simulink model "XecaTurbo_Moist"  (R2023a)
settings: Solver=VariableStepAuto  StartTime=0.0  StopTime=100  RelTol=1e-3  AbsTol=1e-3
PreLoadFcn:
  | omega_TLU = [1000, 1500, 2000, 2500, 3000, 3500];
  | beta_TLU = linspace(0,1,7);
  | 
  | mdot_TLU = [0.1377    0.1304    0.1187    0.1029    0.0854    0.0658    0.0437
  |     0.2310    0.2183    0.1978    0.1688    0.1400    0.1118    0.0750
  |     0.3298    0.3208    0.2987    0.2677    0.2256    0.1774    0.1194
  |     0.4520    0.4260    0.3825    0.3308    0.2745    0.2227    0.1655
  |     0.5542    0.5353    0.4781    0.4230    0.3477    0.2897    0.2211
  |     0.6197    0.5805    0.5198    0.4516    0.3971    0.3555    0.2825];
  | 
  | eta_TLU = [0.7905    0.8025    0.7998    0.7972    0.7932    0.7882    0.7827
  |     0.7993    0.8239    0.8350    0.8379    0.8197    0.8000    0.7809
  |     0.8011    0.8374    0.8632    0.8827    0.8749    0.8394    0.7948
  |     0.8072    0.8520    0.8814    0.9000    0.8676    0.8356    0.7971
  |     0.8076    0.8271    0.8608    0.8766    0.8529    0.8329    0.7992
  |     0.7949    0.8131    0.8296    0.8243    0.8170    0.8085    0.7972];
  | 
  | pr_TLU = [1.0912    1.1795    1.2293    1.2662    1.2928    1.3108    1.3151
  |     1.1484    1.3081    1.3958    1.4707    1.5136    1.5380    1.5456
  |     1.2830    1.4539    1.5943    1.7042    1.7973    1.8582    1.8799
  |     1.5180    1.8034    1.9693    2.0899    2.1662    2.2027    2.2182
  |     1.8359    2.0956    2.3359    2.4668    2.5687    2.6106    2.6224
  |     2.3061    2.6623    2.8585    2.9837    3.0443    3.0714    3.0869];
libraries: nesl_utility x72, fl_lib x52, HVAC_lib x2
(part 1 of 2)
CloseFcn:
  | clear tout simlogCompressorMap
  | clear omega_TLU
  | clear beta_TLU
  | clear mdot_TLU
  | clear pr_TLU
  | clear eta_TLU
Description:
  | Compressor Map
settings Model: Creator=The MathWorks, Inc.  LastModifiedBy=H2FADMIN
settings SolverCC: AutoScaleAbsTol=off  MaxConsecutiveMinStep=25  AlgebraicLoopSolver=TrustRegion  MaxZcPerStep=1
settings DataIOCC: ReturnWorkspaceOutputs=off
settings OptimizationCC: ReuseModelBlockBuffer=off
settings DebuggingCC: UnconnectedInputMsg=warning  UnconnectedOutputMsg=warning  UnconnectedLineMsg=warning  SymbolicDimsDataTypeCodeGenerationDiagnostic=none
settings ModelReferenceCC: EnableRefExpFcnMdlSchedulingChecks=on
settings SFSimCC: CustomCodeUndefinedFunction=UseInterfaceOnly
settings RTWCC: DLArmComputeVersion=19.05
settings SimscapeCC: SimscapeLogType=all  SimscapeLogSimulationStatistics=on  SimscapeLogName=simlogCompressorMap  SimscapeLogDataHistory=10000

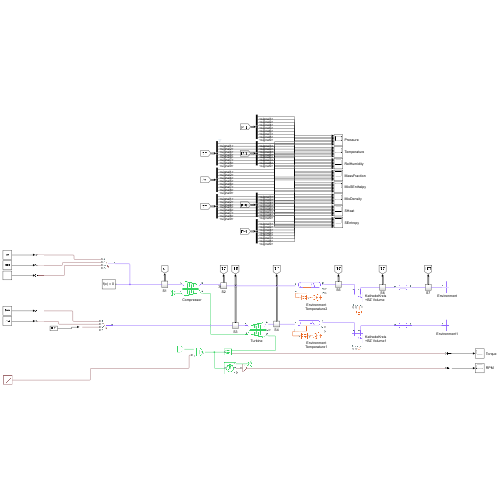
[thumbnail: Simulink's stored preview of the top-level diagram]
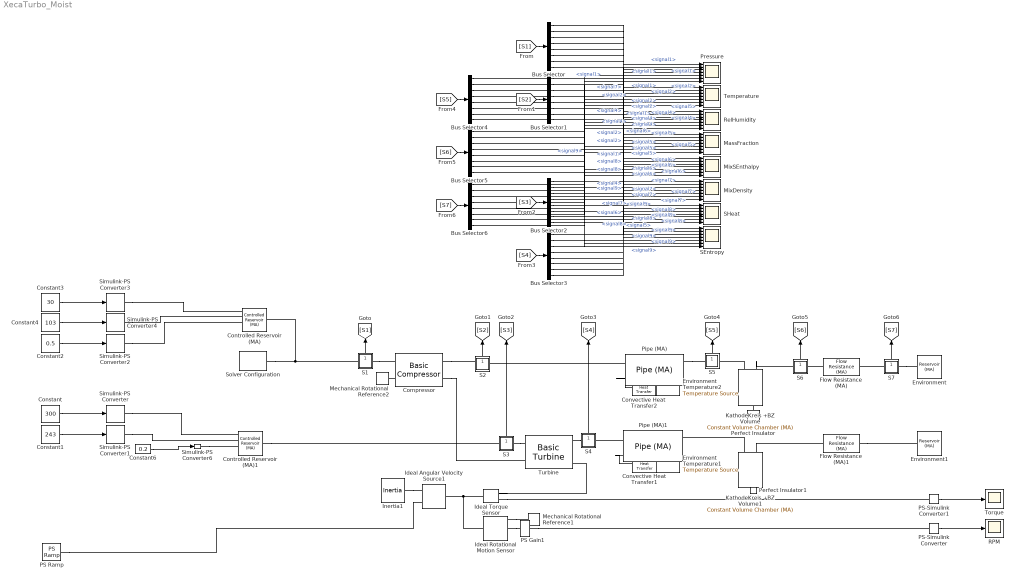
== system XecaTurbo_Moist ==
  Bus Selector{,1..6} (7 alike) : BusSelector  OutputSignals=signal1,signal2,signal4,signal5,signal6,signal7,signal8,signal9
  Compressor : HVAC_lib/Basic Compressor  pr_des=3  mdot_corr_des=.365 kg/s  omega_corr_des=85000 rpm  p_ref=0.101325 MPa  T_ref=288.15 K  RH_ref=0.1  b1=1.5  b2=0.7  b3=0.08  eta_poly=0.95  eta_mech=0.9  area_A=.002 m^2  area_B=.002 m^2
      settings: InternalSimscapePortConfiguration="{\"Bottom\":[],\"Left\":[{\"id\":\"A\",\"label\":\"A\",\"type\":\"foundation.moist_air.moist_air\"},{\"id\":\"C\",\"label\":\"C\",\"type\":\"foundation.mechanical.rotational.rotational\"}],\"Right\":[{\"id\":\"B\",\"label\":\"B\",\"type\":\"foundation.moist_air.moist_air\"},{\"id\":\"R\",\"label\":\"R\",\"type\":\"foundation.mechanical.rotational.rotational\"}],\"Top\":[]}"
  Constant : Constant  Value=300
  Constant1 : Constant  Value=243
  Constant2 : Constant  Value=0.5
  Constant3 : Constant  Value=30
  Constant4 : Constant  Value=103
  Constant6 : Constant  Value=0.2
  Controlled Reservoir (MA) : fl_lib/Moist Air/Elements/Controlled Reservoir (MA)  moisture_spec=foundation.enum.moistureSpec.RelativeHumidity  trace_gas_spec=foundation.enum.trace_gas_spec.mass_fraction  RH_ws=.25  area_A=0.002 m^2  input_error_spec=foundation.enum.input_range_error.limit
      settings: InternalSimscapePortConfiguration="{\"Bottom\":[],\"Left\":[{\"id\":\"A\",\"label\":\"A\",\"type\":\"foundation.moist_air.moist_air\"}],\"Right\":[{\"id\":\"T\",\"label\":\"T\",\"type\":\"input\"},{\"id\":\"P\",\"label\":\"P\",\"type\":\"input\"},{\"id\":\"W\",\"label\":\"W\",\"type\":\"input\"},{\"id\":\"G\",\"label\":\"G\",\"type\":\"input\"}],\"Top\":[]}"
  Controlled Reservoir (MA)1 : fl_lib/Moist Air/Elements/Controlled Reservoir (MA)  moisture_spec=foundation.enum.moistureSpec.RelativeHumidity  trace_gas_spec=foundation.enum.trace_gas_spec.mass_fraction  RH_ws=1  area_A=0.01 m^2  input_error_spec=foundation.enum.input_range_error.limit
      settings: InternalSimscapePortConfiguration="{\"Bottom\":[],\"Left\":[{\"id\":\"A\",\"label\":\"A\",\"type\":\"foundation.moist_air.moist_air\"}],\"Right\":[{\"id\":\"T\",\"label\":\"T\",\"type\":\"input\"},{\"id\":\"P\",\"label\":\"P\",\"type\":\"input\"},{\"id\":\"W\",\"label\":\"W\",\"type\":\"input\"},{\"id\":\"G\",\"label\":\"G\",\"type\":\"input\"}],\"Top\":[]}"
  Convective Heat Transfer1 : fl_lib/Thermal/Thermal Elements/Convective Heat Transfer  thermal_type=foundation.enum.constant_variable.constant  area=.5 m^2  heat_tr_coeff=20 W/(m^2 * K)  min_heat_tr_coeff=1e-3 W/(K*m^2)  T_specify=off  T_priority=None  T=0 K  T_nominal_specify=off  T_nominal_unit=K  T_nominal_value=1  Q_specify=off  Q_priority=None  Q=0 W  Q_nominal_specify=off  Q_nominal_unit=W  Q_nominal_value=1
  Convective Heat Transfer2 : fl_lib/Thermal/Thermal Elements/Convective Heat Transfer  thermal_type=foundation.enum.constant_variable.constant  area=.5 m^2  heat_tr_coeff=20 W/(m^2 * K)  min_heat_tr_coeff=1e-3 W/(K*m^2)  T_specify=off  T_priority=None  T=0 K  T_nominal_specify=off  T_nominal_unit=K  T_nominal_value=1  Q_specify=off  Q_priority=None  Q=0 W  Q_nominal_specify=off  Q_nominal_unit=W  Q_nominal_value=1
  Environment : fl_lib/Moist Air/Elements/Reservoir (MA)  pressure_spec=foundation.enum.pressure_spec.specified  reservoir_pressure=0.103 MPa  temperature_spec=foundation.enum.temperature_spec.specified  reservoir_temperature=20 degC  moisture_spec=foundation.enum.moisture_spec.relative_humidity  reservoir_RH=1  reservoir_x_w=0.01  reservoir_y_w=0.01  reservoir_HR=0.01  reservoir_Tw=287 K  trace_gas_spec=foundation.enum.trace_gas_spec.mole_fraction  reservoir_x_g=0.001  reservoir_y_g=0.1  RH_ws=1  area_A=0.002 m^2
  Environment Temperature1 : fl_lib/Thermal/Thermal Sources/Temperature Source  temperature=20 degC
  Environment Temperature2 : fl_lib/Thermal/Thermal Sources/Temperature Source  temperature=20 degC
  Environment1 : fl_lib/Moist Air/Elements/Reservoir (MA)  pressure_spec=foundation.enum.pressure_spec.specified  reservoir_pressure=0.103 MPa  temperature_spec=foundation.enum.temperature_spec.specified  reservoir_temperature=20 degC  moisture_spec=foundation.enum.moisture_spec.relative_humidity  reservoir_RH=1  reservoir_x_w=0.01  reservoir_y_w=0.01  reservoir_HR=0.01  reservoir_Tw=287 K  trace_gas_spec=foundation.enum.trace_gas_spec.mole_fraction  reservoir_x_g=0.001  reservoir_y_g=0.1  RH_ws=1  area_A=0.002 m^2
  Flow Resistance (MA) : fl_lib/Moist Air/Elements/Flow Resistance (MA)  delta_p_nominal=8 bar  mdot_nominal=.21 kg/s  rho_nominal=3 kg/m^3  area=5.0265482457436691815402294132472e-5 m^2  laminar_fraction=1e-3
  Flow Resistance (MA)1 : fl_lib/Moist Air/Elements/Flow Resistance (MA)  delta_p_nominal=4 bar  mdot_nominal=.21 kg/s  rho_nominal=1.5 kg/m^3  area=5.0265482457436691815402294132472e-5 m^2  laminar_fraction=1e-3
  Ideal Angular Velocity Source1 : fl_lib/Mechanical/Mechanical Sources/Ideal Angular Velocity Source
  Ideal Rotational Motion Sensor : fl_lib/Mechanical/Mechanical Sensors/Ideal Rotational Motion Sensor  reference=foundation.enum.MeasurementReference.difference  acceleration_port=false  velocity_port=true  position_port=true  wrap_angle=false  offset=0 rad
  Ideal Torque Sensor : fl_lib/Mechanical/Mechanical Sensors/Ideal Torque Sensor
  Inertia1 : fl_lib/Mechanical/Rotational Elements/Inertia  inertia=0.03 kg*m^2  num_ports=foundation.enum.numPorts2.one  w_specify=off  w_priority=High  w=0 rad/s  w_nominal_specify=off  w_nominal_unit=rad/s  w_nominal_value=1  t_specify=off  t_priority=None  t=0 N*m  t_nominal_specify=off  t_nominal_unit=N*m  t_nominal_value=1
  KathodeKreis +BZ Volume : fl_lib/Moist Air/Elements/Constant Volume Chamber (MA)  volume=.1 m^3  num_ports=foundation.enum.num_ports.two  area_A=.002 m^2  area_B=.0005 m^2  area_C=0.0005 m^2  area_D=0.01 m^2  RH_ws=1  time_constant=1e-3 s  moisture_trace_gas_source=foundation.enum.moisture_trace_gas_source.controlled  moisture_source_spec=foundation.enum.moisture_source_spec.vapor  moisture_mass_flow=0 kg/s  moisture_temperature_spec=foundation.enum.temperature_spec.atmospheric  moisture_temperature=293.15 K  trace_gas_mass_flow=0 kg/s  trace_gas_temperature_spec=foundation.enum.temperature_spec.atmospheric  trace_gas_temperature=293.15 K  p_I_specify=off  p_I_priority=High  p_I=101.33 kPa  p_I_nominal_specify=off  p_I_nominal_unit=MPa  p_I_nominal_value=1  T_I_specify=off  T_I_priority=High  T_I=45 degC  T_I_nominal_specify=off  T_I_nominal_unit=K  T_I_nominal_value=1  RH_I_specify=off  RH_I_priority=High  RH_I=0.5  RH_I_nominal_specify=off  RH_I_nominal_unit=1  RH_I_nominal_value=1  x_w_I_specify=off  x_w_I_priority=None  x_w_I=0  x_w_I_nominal_specify=off  x_w_I_nominal_unit=1  x_w_I_nominal_value=1  y_w_I_specify=off  y_w_I_priority=None  y_w_I=0  y_w_I_nominal_specify=off  y_w_I_nominal_unit=1  y_w_I_nominal_value=1  HR_I_specify=off  HR_I_priority=None  HR_I=0  HR_I_nominal_specify=off  HR_I_nominal_unit=1  HR_I_nominal_value=1  x_g_I_specify=off  x_g_I_priority=None  x_g_I=0  x_g_I_nominal_specify=off  x_g_I_nominal_unit=1  x_g_I_nominal_value=1  y_g_I_specify=off  y_g_I_priority=High  y_g_I=5e-8  y_g_I_nominal_specify=off  y_g_I_nominal_unit=1  y_g_I_nominal_value=1
      settings: InternalSimscapePortConfiguration="{\"Bottom\":[],\"Left\":[{\"id\":\"A\",\"label\":\"A\",\"type\":\"foundation.moist_air.moist_air\"},{\"id\":\"B\",\"label\":\"B\",\"type\":\"foundation.moist_air.moist_air\"}],\"Right\":[{\"id\":\"W\",\"label\":\"W\",\"type\":\"output\"},{\"id\":\"F\",\"label\":\"F\",\"type\":\"output\"},{\"id\":\"H\",\"label\":\"H\",\"type\":\"foundation.thermal.thermal\"},{\"id\":\"S\",\"label\":\"S\",\"type\":\"foundation.moist_air.moist_air_source\"}],\"Top\":[]}"
  KathodeKreis +BZ Volume1 : fl_lib/Moist Air/Elements/Constant Volume Chamber (MA)  volume=.1 m^3  num_ports=foundation.enum.num_ports.two  area_A=.002 m^2  area_B=.002 m^2  area_C=0.0005 m^2  area_D=0.01 m^2  RH_ws=1  time_constant=1e-3 s  moisture_trace_gas_source=foundation.enum.moisture_trace_gas_source.controlled  moisture_source_spec=foundation.enum.moisture_source_spec.vapor  moisture_mass_flow=0 kg/s  moisture_temperature_spec=foundation.enum.temperature_spec.atmospheric  moisture_temperature=293.15 K  trace_gas_mass_flow=0 kg/s  trace_gas_temperature_spec=foundation.enum.temperature_spec.atmospheric  trace_gas_temperature=293.15 K  p_I_specify=off  p_I_priority=High  p_I=101.33 kPa  p_I_nominal_specify=off  p_I_nominal_unit=MPa  p_I_nominal_value=1  T_I_specify=on  T_I_priority=High  T_I=45 degC  T_I_nominal_specify=off  T_I_nominal_unit=K  T_I_nominal_value=1  RH_I_specify=off  RH_I_priority=High  RH_I=0.5  RH_I_nominal_specify=off  RH_I_nominal_unit=1  RH_I_nominal_value=1  x_w_I_specify=off  x_w_I_priority=None  x_w_I=0  x_w_I_nominal_specify=off  x_w_I_nominal_unit=1  x_w_I_nominal_value=1  y_w_I_specify=off  y_w_I_priority=None  y_w_I=0  y_w_I_nominal_specify=off  y_w_I_nominal_unit=1  y_w_I_nominal_value=1  HR_I_specify=off  HR_I_priority=None  HR_I=0  HR_I_nominal_specify=off  HR_I_nominal_unit=1  HR_I_nominal_value=1  x_g_I_specify=off  x_g_I_priority=None  x_g_I=0  x_g_I_nominal_specify=off  x_g_I_nominal_unit=1  x_g_I_nominal_value=1  y_g_I_specify=off  y_g_I_priority=High  y_g_I=5e-8  y_g_I_nominal_specify=off  y_g_I_nominal_unit=1  y_g_I_nominal_value=1
      settings: InternalSimscapePortConfiguration="{\"Bottom\":[],\"Left\":[{\"id\":\"A\",\"label\":\"A\",\"type\":\"foundation.moist_air.moist_air\"},{\"id\":\"B\",\"label\":\"B\",\"type\":\"foundation.moist_air.moist_air\"}],\"Right\":[{\"id\":\"W\",\"label\":\"W\",\"type\":\"output\"},{\"id\":\"F\",\"label\":\"F\",\"type\":\"output\"},{\"id\":\"H\",\"label\":\"H\",\"type\":\"foundation.thermal.thermal\"},{\"id\":\"S\",\"label\":\"S\",\"type\":\"foundation.moist_air.moist_air_source\"}],\"Top\":[]}"
  MassFraction : Scope  NumInputPorts=7
  Mechanical Rotational Reference1 : fl_lib/Mechanical/Rotational Elements/Mechanical Rotational Reference
  Mechanical Rotational Reference2 : fl_lib/Mechanical/Rotational Elements/Mechanical Rotational Reference
  MixDensity : Scope  NumInputPorts=7
  MixSEnthalpy : Scope  NumInputPorts=7
  PS Gain1 : fl_lib/Physical Signals/Functions/PS Gain  gain=1/(0.1047198*1000)
  PS Ramp : fl_lib/Physical Signals/Sources/PS Ramp  slope=(85000-31000)/90 rpm/s  start_time=10 s  initial_output=31000 rpm
  PS-Simulink Converter : nesl_utility/PS-Simulink Converter  PhysicalDomain=network_engine_domain  SubClassName=ps_output  LeftPortType=input  RightPortType=output  PseudoPeriodic=off  Frequencies=[]  VectorFormat=inherit  Unit=inherit  AffineConversion=off
  PS-Simulink Converter1 : nesl_utility/PS-Simulink Converter  PhysicalDomain=network_engine_domain  SubClassName=ps_output  LeftPortType=input  RightPortType=output  PseudoPeriodic=off  Frequencies=[]  VectorFormat=inherit  Unit=inherit  AffineConversion=off
  Perfect Insulator : fl_lib/Thermal/Thermal Elements/Perfect Insulator  T_specify=off  T_priority=None  T=293.15 K  T_nominal_specify=off  T_nominal_unit=K  T_nominal_value=1
  Perfect Insulator1 : fl_lib/Thermal/Thermal Elements/Perfect Insulator  T_specify=off  T_priority=None  T=293.15 K  T_nominal_specify=off  T_nominal_unit=K  T_nominal_value=1
  Pipe (MA) : fl_lib/Moist Air/Elements/Pipe (MA)  length=1 m  area=.002 m^2  Dh=.1 m  length_add=1 m  roughness=15e-5 m  Re_lam=2000  Re_tur=4000  shape_factor=64  Nu_lam=3.66  wall_condensation=simscape.enum.onoff.off  RH_ws=1  time_constant=1e-3 s  moisture_trace_gas_source=foundation.enum.moisture_trace_gas_source.none  moisture_source_spec=foundation.enum.moisture_source_spec.vapor  moisture_mass_flow=0 kg/s  moisture_temperature_spec=foundation.enum.temperature_spec.atmospheric  moisture_temperature=293.15 K  trace_gas_mass_flow=0 kg/s  trace_gas_temperature_spec=foundation.enum.temperature_spec.atmospheric  trace_gas_temperature=293.15 K  p_I_specify=off  p_I_priority=High  p_I=0.103 MPa  p_I_nominal_specify=off  p_I_nominal_unit=MPa  p_I_nominal_value=1  T_I_specify=off  T_I_priority=High  T_I=20 degC  T_I_nominal_specify=off  T_I_nominal_unit=K  T_I_nominal_value=1  RH_I_specify=off  RH_I_priority=High  RH_I=1  RH_I_nominal_specify=off  RH_I_nominal_unit=1  RH_I_nominal_value=1  x_w_I_specify=off  x_w_I_priority=None  x_w_I=0  x_w_I_nominal_specify=off  x_w_I_nominal_unit=1  x_w_I_nominal_value=1  y_w_I_specify=off  y_w_I_priority=None  y_w_I=0  y_w_I_nominal_specify=off  y_w_I_nominal_unit=1  y_w_I_nominal_value=1  HR_I_specify=off  HR_I_priority=None  HR_I=0  HR_I_nominal_specify=off  HR_I_nominal_unit=1  HR_I_nominal_value=1  x_g_I_specify=off  x_g_I_priority=None  x_g_I=0  x_g_I_nominal_specify=off  x_g_I_nominal_unit=1  x_g_I_nominal_value=1  y_g_I_specify=off  y_g_I_priority=High  y_g_I=0.1  y_g_I_nominal_specify=off  y_g_I_nominal_unit=1  y_g_I_nominal_value=1
  Pipe (MA)1 : fl_lib/Moist Air/Elements/Pipe (MA)  length=1 m  area=.002 m^2  Dh=.1 m  length_add=1 m  roughness=15e-5 m  Re_lam=2000  Re_tur=4000  shape_factor=64  Nu_lam=3.66  wall_condensation=simscape.enum.onoff.off  RH_ws=1  time_constant=1e-3 s  moisture_trace_gas_source=foundation.enum.moisture_trace_gas_source.none  moisture_source_spec=foundation.enum.moisture_source_spec.vapor  moisture_mass_flow=0 kg/s  moisture_temperature_spec=foundation.enum.temperature_spec.atmospheric  moisture_temperature=293.15 K  trace_gas_mass_flow=0 kg/s  trace_gas_temperature_spec=foundation.enum.temperature_spec.atmospheric  trace_gas_temperature=293.15 K  p_I_specify=off  p_I_priority=High  p_I=0.103 MPa  p_I_nominal_specify=off  p_I_nominal_unit=MPa  p_I_nominal_value=1  T_I_specify=off  T_I_priority=High  T_I=20 degC  T_I_nominal_specify=off  T_I_nominal_unit=K  T_I_nominal_value=1  RH_I_specify=off  RH_I_priority=High  RH_I=1  RH_I_nominal_specify=off  RH_I_nominal_unit=1  RH_I_nominal_value=1  x_w_I_specify=off  x_w_I_priority=None  x_w_I=0  x_w_I_nominal_specify=off  x_w_I_nominal_unit=1  x_w_I_nominal_value=1  y_w_I_specify=off  y_w_I_priority=None  y_w_I=0  y_w_I_nominal_specify=off  y_w_I_nominal_unit=1  y_w_I_nominal_value=1  HR_I_specify=off  HR_I_priority=None  HR_I=0  HR_I_nominal_specify=off  HR_I_nominal_unit=1  HR_I_nominal_value=1  x_g_I_specify=off  x_g_I_priority=None  x_g_I=0  x_g_I_nominal_specify=off  x_g_I_nominal_unit=1  x_g_I_nominal_value=1  y_g_I_specify=off  y_g_I_priority=High  y_g_I=0.1  y_g_I_nominal_specify=off  y_g_I_nominal_unit=1  y_g_I_nominal_value=1
  Pressure : Scope  NumInputPorts=7
  RPM : Scope
  RelHumidity : Scope  NumInputPorts=7
  S1 : Subsystem
      settings: PortSchema="{\"entries\":[{\"content\":{\"sides\":[{\"content\":{\"connectorIds\":[\"LConn1\"]},\"type\":\"ConnectorPlacement.EquallySpacedRectSide\",\"uuid\":\"254e2835-1051-41ce-ae2c-1054ced4b7e5\"},{\"content\":{\"connectorIds\":[\"RConn1\"],\"side\":\"RIGHT\"},\"type\":\"ConnectorPlacement.EquallySpacedRectSide\",\"uuid\":\"319e61c8-525d-4586-8cb8-060a189dde36\"},{\"content\":{\"connectorIds\":[\"Out1\"],\"side\":\"TOP\"},\"type\":\"ConnectorPlacement.EquallySpacedRectSide\",\"uuid\":\"621e15c0-a15c-4528-a2f1-5cf6f15ed99c\"}]},\"type\":\"ConnectorPlacement.EquallySpacedConnector\",\"uuid\":\"0cef8054-f5e2-4319-9020-84a4d4054be4\"}],\"packageUris\":[\"http://schema.mathworks.com/mf0/Connector/R2020b\"],\"version\":\"1.0\"}"
  S2 : Subsystem
      settings: PortSchema="{\"entries\":[{\"content\":{\"sides\":[{\"content\":{\"connectorIds\":[\"LConn1\",\"LConn2\",\"LConn3\"]},\"type\":\"ConnectorPlacement.EquallySpacedRectSide\",\"uuid\":\"2c3dff3d-006a-434f-af42-26af1dfa59bd\"},{\"content\":{\"connectorIds\":[\"RConn1\"],\"side\":\"RIGHT\"},\"type\":\"ConnectorPlacement.EquallySpacedRectSide\",\"uuid\":\"5c8d4e8e-dace-4a30-a25f-c68d34fe03f2\"},{\"content\":{\"connectorIds\":[\"Out1\"],\"side\":\"TOP\"},\"type\":\"ConnectorPlacement.EquallySpacedRectSide\",\"uuid\":\"01211e8f-380a-4edd-8d10-28a378ec8de7\"}]},\"type\":\"ConnectorPlacement.EquallySpacedConnector\",\"uuid\":\"cc392eb8-3a05-4333-a2d0-35104579f5e5\"}],\"packageUris\":[\"http://schema.mathworks.com/mf0/Connector/R2020b\"],\"version\":\"1.0\"}"
  S3 : Subsystem
      settings: PortSchema="{\"entries\":[{\"content\":{\"sides\":[{\"content\":{\"connectorIds\":[\"LConn1\"]},\"type\":\"ConnectorPlacement.EquallySpacedRectSide\",\"uuid\":\"254e2835-1051-41ce-ae2c-1054ced4b7e5\"},{\"content\":{\"connectorIds\":[\"RConn1\"],\"side\":\"RIGHT\"},\"type\":\"ConnectorPlacement.EquallySpacedRectSide\",\"uuid\":\"319e61c8-525d-4586-8cb8-060a189dde36\"},{\"content\":{\"connectorIds\":[\"Out1\"],\"side\":\"TOP\"},\"type\":\"ConnectorPlacement.EquallySpacedRectSide\",\"uuid\":\"621e15c0-a15c-4528-a2f1-5cf6f15ed99c\"}]},\"type\":\"ConnectorPlacement.EquallySpacedConnector\",\"uuid\":\"0cef8054-f5e2-4319-9020-84a4d4054be4\"}],\"packageUris\":[\"http://schema.mathworks.com/mf0/Connector/R2020b\"],\"version\":\"1.0\"}"
  S4 : Subsystem
      settings: PortSchema="{\"entries\":[{\"content\":{\"sides\":[{\"content\":{\"connectorIds\":[\"LConn1\"]},\"type\":\"ConnectorPlacement.EquallySpacedRectSide\",\"uuid\":\"254e2835-1051-41ce-ae2c-1054ced4b7e5\"},{\"content\":{\"connectorIds\":[\"RConn1\"],\"side\":\"RIGHT\"},\"type\":\"ConnectorPlacement.EquallySpacedRectSide\",\"uuid\":\"319e61c8-525d-4586-8cb8-060a189dde36\"},{\"content\":{\"connectorIds\":[\"Out1\"],\"side\":\"TOP\"},\"type\":\"ConnectorPlacement.EquallySpacedRectSide\",\"uuid\":\"621e15c0-a15c-4528-a2f1-5cf6f15ed99c\"}]},\"type\":\"ConnectorPlacement.EquallySpacedConnector\",\"uuid\":\"0cef8054-f5e2-4319-9020-84a4d4054be4\"}],\"packageUris\":[\"http://schema.mathworks.com/mf0/Connector/R2020b\"],\"version\":\"1.0\"}"
  S5 : Subsystem
      settings: PortSchema="{\"entries\":[{\"content\":{\"sides\":[{\"content\":{\"connectorIds\":[\"LConn1\"]},\"type\":\"ConnectorPlacement.EquallySpacedRectSide\",\"uuid\":\"254e2835-1051-41ce-ae2c-1054ced4b7e5\"},{\"content\":{\"connectorIds\":[\"RConn1\"],\"side\":\"RIGHT\"},\"type\":\"ConnectorPlacement.EquallySpacedRectSide\",\"uuid\":\"319e61c8-525d-4586-8cb8-060a189dde36\"},{\"content\":{\"connectorIds\":[\"Out1\"],\"side\":\"TOP\"},\"type\":\"ConnectorPlacement.EquallySpacedRectSide\",\"uuid\":\"621e15c0-a15c-4528-a2f1-5cf6f15ed99c\"}]},\"type\":\"ConnectorPlacement.EquallySpacedConnector\",\"uuid\":\"0cef8054-f5e2-4319-9020-84a4d4054be4\"}],\"packageUris\":[\"http://schema.mathworks.com/mf0/Connector/R2020b\"],\"version\":\"1.0\"}"
  S6 : Subsystem
      settings: PortSchema="{\"entries\":[{\"content\":{\"sides\":[{\"content\":{\"connectorIds\":[\"LConn1\"]},\"type\":\"ConnectorPlacement.EquallySpacedRectSide\",\"uuid\":\"254e2835-1051-41ce-ae2c-1054ced4b7e5\"},{\"content\":{\"connectorIds\":[\"RConn1\"],\"side\":\"RIGHT\"},\"type\":\"ConnectorPlacement.EquallySpacedRectSide\",\"uuid\":\"319e61c8-525d-4586-8cb8-060a189dde36\"},{\"content\":{\"connectorIds\":[\"Out1\"],\"side\":\"TOP\"},\"type\":\"ConnectorPlacement.EquallySpacedRectSide\",\"uuid\":\"621e15c0-a15c-4528-a2f1-5cf6f15ed99c\"}]},\"type\":\"ConnectorPlacement.EquallySpacedConnector\",\"uuid\":\"0cef8054-f5e2-4319-9020-84a4d4054be4\"}],\"packageUris\":[\"http://schema.mathworks.com/mf0/Connector/R2020b\"],\"version\":\"1.0\"}"
  S7 : Subsystem
      settings: PortSchema="{\"entries\":[{\"content\":{\"sides\":[{\"content\":{\"connectorIds\":[\"LConn1\"]},\"type\":\"ConnectorPlacement.EquallySpacedRectSide\",\"uuid\":\"254e2835-1051-41ce-ae2c-1054ced4b7e5\"},{\"content\":{\"connectorIds\":[\"RConn1\"],\"side\":\"RIGHT\"},\"type\":\"ConnectorPlacement.EquallySpacedRectSide\",\"uuid\":\"319e61c8-525d-4586-8cb8-060a189dde36\"},{\"content\":{\"connectorIds\":[\"Out1\"],\"side\":\"TOP\"},\"type\":\"ConnectorPlacement.EquallySpacedRectSide\",\"uuid\":\"621e15c0-a15c-4528-a2f1-5cf6f15ed99c\"}]},\"type\":\"ConnectorPlacement.EquallySpacedConnector\",\"uuid\":\"0cef8054-f5e2-4319-9020-84a4d4054be4\"}],\"packageUris\":[\"http://schema.mathworks.com/mf0/Connector/R2020b\"],\"version\":\"1.0\"}"
  SEntropy : Scope  NumInputPorts=7
  SHeat : Scope  NumInputPorts=7
  Simulink-PS Converter : nesl_utility/Simulink-PS Converter  PhysicalDomain=network_engine_domain  SubClassName=ps_input  LeftPortType=input  RightPortType=output  PseudoPeriodic=off  Frequencies=[]  NoiseDistribution=none  NoiseParameters=[]  Unit=degC  AffineConversion=off  FilteringAndDerivatives=provide  SimscapeFilterOrder=1  InputFilterTimeConstant=0.001  UdotUserProvided=0
  Simulink-PS Converter1 : nesl_utility/Simulink-PS Converter  PhysicalDomain=network_engine_domain  SubClassName=ps_input  LeftPortType=input  RightPortType=output  PseudoPeriodic=off  Frequencies=[]  NoiseDistribution=none  NoiseParameters=[]  Unit=kPa  AffineConversion=off  FilteringAndDerivatives=provide  SimscapeFilterOrder=1  InputFilterTimeConstant=0.001  UdotUserProvided=0
  Simulink-PS Converter2 : nesl_utility/Simulink-PS Converter  PhysicalDomain=network_engine_domain  SubClassName=ps_input  LeftPortType=input  RightPortType=output  PseudoPeriodic=off  Frequencies=[]  NoiseDistribution=none  NoiseParameters=[]  Unit=1  AffineConversion=off  FilteringAndDerivatives=provide  SimscapeFilterOrder=1  InputFilterTimeConstant=0.001  UdotUserProvided=0
  Simulink-PS Converter3 : nesl_utility/Simulink-PS Converter  PhysicalDomain=network_engine_domain  SubClassName=ps_input  LeftPortType=input  RightPortType=output  PseudoPeriodic=off  Frequencies=[]  NoiseDistribution=none  NoiseParameters=[]  Unit=degC  AffineConversion=off  FilteringAndDerivatives=provide  SimscapeFilterOrder=1  InputFilterTimeConstant=0.001  UdotUserProvided=0
  Simulink-PS Converter4 : nesl_utility/Simulink-PS Converter  PhysicalDomain=network_engine_domain  SubClassName=ps_input  LeftPortType=input  RightPortType=output  PseudoPeriodic=off  Frequencies=[]  NoiseDistribution=none  NoiseParameters=[]  Unit=kPa  AffineConversion=off  FilteringAndDerivatives=provide  SimscapeFilterOrder=1  InputFilterTimeConstant=0.001  UdotUserProvided=0
  Simulink-PS Converter6 : nesl_utility/Simulink-PS Converter  PhysicalDomain=network_engine_domain  SubClassName=ps_input  LeftPortType=input  RightPortType=output  PseudoPeriodic=off  Frequencies=[]  NoiseDistribution=none  NoiseParameters=[]  Unit=1  AffineConversion=off  FilteringAndDerivatives=provide  SimscapeFilterOrder=1  InputFilterTimeConstant=0.001  UdotUserProvided=0
  Solver Configuration : nesl_utility/Solver Configuration  PhysicalDomain=network_engine_domain  SubClassName=solver  LeftPortType=input  RightPortType=generic  Tones=[]  Harmonics=[]  SimulateNoise=off  Profile=off  UseLocalSampling=off  EnableSwitchedLinearOptims=on  FrequencyDomain=off  UseCCode=off  RelTol=0.001  AbsTol=0.001  MinStep=1e-09  ToWorkspace=off  RevertToSquareIcSolve=off  NumHomotopyIterations=100  PhasorMode=off  PhasorModeNumHarmonics=1  ConsistencySolver=NEWTON_XTOL_AFTER_FTOL  IndexReductionMethod=DerivativeReplacement  DoDC=off  ResidualTolerance=1e-09  ConsistencyTolSource=GLOBAL  ConsistencyAbsTol=0.001  ConsistencyRelTol=0.001  ConsistencyTolFactor=0.001  UseLocalSolver=on  LocalSolverChoice=NE_BACKWARD_EULER_ADVANCER  ResolveIndetEquations=on  FunctionEvalNumThread=1  LocalSolverSampleTime=0.001  DoFixedCost=on  MaxNonlinIter=3  MaxModeIter=2  ComputeImpulses=off  ImpulseIterations=2  LinearAlgebra=auto  LinearAlgebraNumThread=0  EquationFormulation=NE_TIME_EF  DelaysMemoryBudget=1024  AutomaticFiltering=on  FilteringTimeConstant=0.001  PartitionStorageMethod=AS_NEEDED  PartitionMemoryBudget=1024  PartitionMethod=ROBUST
  Temperature : Scope  NumInputPorts=7
  Torque : Scope
  Turbine : HVAC_lib/Basic Turbine  pr_des=0.2  mdot_corr_des=0.22 kg/s  p_ref=0.101325 MPa  T_ref=288.15 K  RH_ref=0  eta_poly=0.92  eta_mech=0.98  area_A=.002 m^2  area_B=.002 m^2  RH_ws=1
      settings: InternalSimscapePortConfiguration="{\"Bottom\":[],\"Left\":[{\"id\":\"A\",\"label\":\"A\",\"type\":\"foundation.moist_air.moist_air\"},{\"id\":\"R\",\"label\":\"R\",\"type\":\"foundation.mechanical.rotational.rotational\"}],\"Right\":[{\"id\":\"B\",\"label\":\"B\",\"type\":\"foundation.moist_air.moist_air\"},{\"id\":\"W\",\"label\":\"W\",\"type\":\"output\"},{\"id\":\"C\",\"label\":\"C\",\"type\":\"foundation.mechanical.rotational.rotational\"}],\"Top\":[]}"
  wires:
  Bus Selector3/2 -> Temperature/4  "<signal2>"
  Bus Selector2/8 -> SEntropy/3  "<signal9>"
  [S1] -> Bus Selector/1
  Bus Selector3/4 -> MassFraction/4  "<signal5>"
  Bus Selector1/7 -> SHeat/2  "<signal8>"
  Bus Selector1/6 -> MixDensity/2  "<signal7>"
  [S2] -> Bus Selector1/1
  Bus Selector4/2 -> Temperature/6  "<signal2>"
  Bus Selector5/3 -> RelHumidity/5  "<signal4>"
  PS-Simulink Converter/1 -> RPM/1
  [S3] -> Bus Selector2/1
  Bus Selector5/4 -> MassFraction/5  "<signal5>"
  [S6] -> Bus Selector5/1
  [S4] -> Bus Selector3/1
  [S5] -> Bus Selector4/1
  [S7] -> Bus Selector6/1
  Bus Selector6/1 -> Pressure/7  "<signal1>"
  Bus Selector1/2 -> Temperature/2  "<signal2>"
  Bus Selector2/5 -> MixSEnthalpy/3  "<signal6>"
  S1/1(Outport) -> [S1]
  Bus Selector/2 -> Temperature/1  "<signal2>"
  Bus Selector/1 -> Pressure/1  "<signal1>"
  Bus Selector/4 -> RelHumidity/1  "<signal5>"
  Bus Selector5/1 -> Pressure/5  "<signal1>"
  Bus Selector/3 -> MassFraction/1  "<signal4>"
  Bus Selector1/5 -> MixSEnthalpy/2  "<signal6>"
  Bus Selector/5 -> MixSEnthalpy/1  "<signal6>"
  Bus Selector/8 -> SEntropy/1  "<signal9>"
  Bus Selector/6 -> MixDensity/1  "<signal7>"
  Bus Selector/7 -> SHeat/1  "<signal8>"
  Bus Selector1/1 -> Pressure/2  "<signal1>"
  Bus Selector4/4 -> MassFraction/6  "<signal5>"
  Bus Selector5/6 -> MixDensity/5  "<signal7>"
  Bus Selector3/7 -> SHeat/4  "<signal8>"
  Bus Selector1/3 -> RelHumidity/2  "<signal4>"
  Bus Selector1/4 -> MassFraction/2  "<signal5>"
  Bus Selector2/2 -> Temperature/3  "<signal2>"
  Bus Selector1/8 -> SEntropy/2  "<signal9>"
  Bus Selector2/1 -> Pressure/3  "<signal1>"
  Bus Selector2/3 -> RelHumidity/3  "<signal4>"
  Bus Selector2/4 -> MassFraction/3  "<signal5>"
  Bus Selector2/6 -> MixDensity/3  "<signal7>"
  Bus Selector2/7 -> SHeat/3  "<signal8>"
  Bus Selector3/1 -> Pressure/4  "<signal1>"
  Bus Selector4/3 -> RelHumidity/6  "<signal4>"
  Bus Selector3/3 -> RelHumidity/4  "<signal4>"
  Bus Selector3/5 -> MixSEnthalpy/4  "<signal6>"
  Bus Selector3/6 -> MixDensity/4  "<signal7>"
  Bus Selector3/8 -> SEntropy/4  "<signal9>"
  Bus Selector4/1 -> Pressure/6  "<signal1>"
  Bus Selector5/2 -> Temperature/5  "<signal2>"
  Bus Selector5/5 -> MixSEnthalpy/5  "<signal6>"
  Bus Selector4/5 -> MixSEnthalpy/6  "<signal6>"
  Bus Selector5/7 -> SHeat/5  "<signal8>"
  Bus Selector4/6 -> MixDensity/6  "<signal7>"
  Bus Selector5/8 -> SEntropy/5  "<signal9>"
  Bus Selector4/7 -> SHeat/6  "<signal8>"
  Bus Selector4/8 -> SEntropy/6  "<signal9>"
  Bus Selector6/2 -> Temperature/7  "<signal2>"
  Bus Selector6/3 -> RelHumidity/7  "<signal4>"
  Bus Selector6/4 -> MassFraction/7  "<signal5>"
  Bus Selector6/5 -> MixSEnthalpy/7  "<signal6>"
  Bus Selector6/6 -> MixDensity/7  "<signal7>"
  Bus Selector6/7 -> SHeat/7  "<signal8>"
  Bus Selector6/8 -> SEntropy/7  "<signal9>"
  PS-Simulink Converter1/1 -> Torque/1
  S2/1(Outport) -> [S2]
  S3/1(Outport) -> [S3]
  S4/1(Outport) -> [S4]
  S5/1(Outport) -> [S5]
  S6/1(Outport) -> [S6]
  S7/1(Outport) -> [S7]
  Constant2/1 -> Simulink-PS Converter2/1
  Constant/1 -> Simulink-PS Converter/1
  Constant1/1 -> Simulink-PS Converter1/1
  Constant6/1 -> Simulink-PS Converter6/1
  Constant4/1 -> Simulink-PS Converter4/1
  Constant3/1 -> Simulink-PS Converter3/1
  connections:
  Ideal Rotational Motion Sensor/RConn2 -- PS Gain1/LConn1
  Ideal Rotational Motion Sensor/RConn1 -- Mechanical Rotational Reference1/LConn1
  Ideal Torque Sensor/RConn2 -- PS-Simulink Converter1/LConn1
  Inertia1/LConn1 -- Ideal Angular Velocity Source1/RConn2
  Ideal Rotational Motion Sensor/LConn1 -- Ideal Torque Sensor/LConn1 -- Ideal Angular Velocity Source1/LConn1
  PS Ramp/RConn1 -- Ideal Angular Velocity Source1/RConn1
  Solver Configuration/RConn1 -- S1/LConn1 -- Controlled Reservoir (MA)/LConn1
  PS Gain1/RConn1 -- PS-Simulink Converter/LConn1
  S1/RConn1 -- Compressor/LConn1
  KathodeKreis +BZ Volume/LConn2 -- S6/LConn1
  Compressor/RConn2 -- Turbine/LConn2
  Compressor/RConn1 -- S2/LConn1
  Controlled Reservoir (MA)1/LConn1 -- S3/LConn1
  S3/RConn1 -- Turbine/LConn1
  Turbine/RConn1 -- S4/LConn1
  Ideal Torque Sensor/RConn1 -- Turbine/RConn3
  KathodeKreis +BZ Volume/LConn1 -- S5/RConn1
  Pipe (MA)/LConn2 -- Convective Heat Transfer2/LConn1
  Flow Resistance (MA)/LConn1 -- S6/RConn1
  Convective Heat Transfer2/RConn1 -- Environment Temperature2/LConn1
  Pipe (MA)/RConn1 -- S5/LConn1
  Simulink-PS Converter3/RConn1 -- Controlled Reservoir (MA)/RConn1
  Simulink-PS Converter4/RConn1 -- Controlled Reservoir (MA)/RConn2
  Simulink-PS Converter2/RConn1 -- Controlled Reservoir (MA)/RConn3
  Simulink-PS Converter6/RConn1 -- Controlled Reservoir (MA)1/RConn3
  S7/LConn1 -- Flow Resistance (MA)/RConn1
  S7/RConn1 -- Environment/LConn1
  Perfect Insulator/LConn1 -- KathodeKreis +BZ Volume/RConn3
  Pipe (MA)/LConn1 -- S2/RConn1
  Perfect Insulator1/LConn1 -- KathodeKreis +BZ Volume1/RConn3
  Convective Heat Transfer1/RConn1 -- Environment Temperature1/LConn1
  Flow Resistance (MA)1/RConn1 -- Environment1/LConn1
  KathodeKreis +BZ Volume1/LConn2 -- Flow Resistance (MA)1/LConn1
  Pipe (MA)1/LConn1 -- S4/RConn1
  Pipe (MA)1/LConn2 -- Convective Heat Transfer1/LConn1
  KathodeKreis +BZ Volume1/LConn1 -- Pipe (MA)1/RConn1
  Simulink-PS Converter/RConn1 -- Controlled Reservoir (MA)1/RConn1
  Simulink-PS Converter1/RConn1 -- Controlled Reservoir (MA)1/RConn2
  Mechanical Rotational Reference2/LConn1 -- Compressor/LConn2

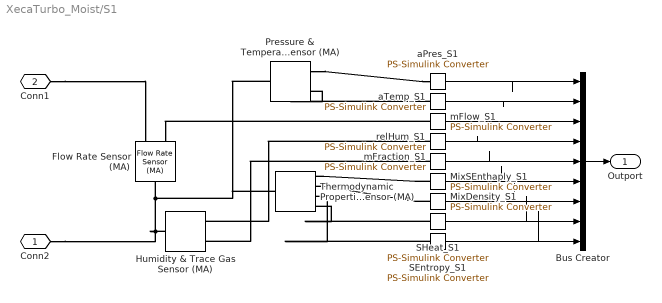
== system XecaTurbo_Moist/S1 ==
  Bus Creator : BusCreator  Inputs=9
  Flow Rate Sensor (MA) : fl_lib/Moist Air/Sensors/Flow Rate Sensor (MA)  mass_flow_measure=true  volumetric_flow_measure=false  volumetric_flow_conditions=foundation.enum.volumetric_flow_conditions.actual  p_std=0.101325 MPa  T_std=20 degC  RH_std=0.65  energy_flow_measure=false  vapor_flow_measure=false  gas_flow_measure=false
      settings: InternalSimscapePortConfiguration="{\"Bottom\":[],\"Left\":[{\"id\":\"A\",\"label\":\"A\",\"type\":\"foundation.moist_air.moist_air\"}],\"Right\":[{\"id\":\"B\",\"label\":\"B\",\"type\":\"foundation.moist_air.moist_air\"},{\"id\":\"M\",\"label\":\"M\",\"type\":\"output\"}],\"Top\":[]}"
  Humidity & Trace Gas Sensor (MA) : fl_lib/Moist Air/Sensors/Humidity & Trace Gas Sensor (MA)  moisture_on=true  moisture_spec=foundation.enum.moistureSpec.SpecificHumidity  trace_gas_on=true  trace_gas_spec=foundation.enum.trace_gas_spec.mass_fraction
      settings: InternalSimscapePortConfiguration="{\"Bottom\":[],\"Left\":[{\"id\":\"A\",\"label\":\"A\",\"type\":\"foundation.moist_air.moist_air\"}],\"Right\":[{\"id\":\"W\",\"label\":\"W\",\"type\":\"output\"},{\"id\":\"G\",\"label\":\"G\",\"type\":\"output\"}],\"Top\":[]}"
  MixDensity_S1 : nesl_utility/PS-Simulink Converter  PhysicalDomain=network_engine_domain  SubClassName=ps_output  LeftPortType=input  RightPortType=output  PseudoPeriodic=off  Frequencies=[]  VectorFormat=inherit  Unit=inherit  AffineConversion=off
  MixSEnthaply_S1 : nesl_utility/PS-Simulink Converter  PhysicalDomain=network_engine_domain  SubClassName=ps_output  LeftPortType=input  RightPortType=output  PseudoPeriodic=off  Frequencies=[]  VectorFormat=inherit  Unit=inherit  AffineConversion=off
  Pressure & Temperature Sensor (MA) : fl_lib/Moist Air/Sensors/Pressure & Temperature Sensor (MA)  reference=foundation.enum.MeasurementReference.absolute  pressure=true  pressure_spec=foundation.enum.PressureMeasementSpec.Absolute  temperature=true
      settings: InternalSimscapePortConfiguration="{\"Bottom\":[{\"id\":\"T\",\"label\":\"T\",\"type\":\"output\"}],\"Left\":[{\"id\":\"A\",\"label\":\"A\",\"type\":\"foundation.moist_air.moist_air\"}],\"Right\":[{\"id\":\"Pa\",\"label\":\"Pa\",\"type\":\"output\"}],\"Top\":[]}"
  SEntropy_S1 : nesl_utility/PS-Simulink Converter  PhysicalDomain=network_engine_domain  SubClassName=ps_output  LeftPortType=input  RightPortType=output  PseudoPeriodic=off  Frequencies=[]  VectorFormat=inherit  Unit=inherit  AffineConversion=off
  SHeat_S1 : nesl_utility/PS-Simulink Converter  PhysicalDomain=network_engine_domain  SubClassName=ps_output  LeftPortType=input  RightPortType=output  PseudoPeriodic=off  Frequencies=[]  VectorFormat=inherit  Unit=inherit  AffineConversion=off
  Thermodynamic Properties Sensor (MA) : fl_lib/Moist Air/Sensors/Thermodynamic Properties Sensor (MA)  measurement_mass_spec=foundation.enum.measurement_mass_spec.mixture  enthalpy=true  density=true  specific_heat=true  entropy=true
      settings: InternalSimscapePortConfiguration="{\"Bottom\":[{\"id\":\"CP\",\"label\":\"cp\",\"type\":\"output\"},{\"id\":\"S\",\"label\":\"s\",\"type\":\"output\"}],\"Left\":[{\"id\":\"A\",\"label\":\"A\",\"type\":\"foundation.moist_air.moist_air\"}],\"Right\":[{\"id\":\"H\",\"label\":\"h\",\"type\":\"output\"},{\"id\":\"RHO\",\"label\":\"ρ\",\"type\":\"output\"}],\"Top\":[]}"
  aPres_S1 : nesl_utility/PS-Simulink Converter  PhysicalDomain=network_engine_domain  SubClassName=ps_output  LeftPortType=input  RightPortType=output  PseudoPeriodic=off  Frequencies=[]  VectorFormat=inherit  Unit=inherit  AffineConversion=off
  aTemp_S1 : nesl_utility/PS-Simulink Converter  PhysicalDomain=network_engine_domain  SubClassName=ps_output  LeftPortType=input  RightPortType=output  PseudoPeriodic=off  Frequencies=[]  VectorFormat=inherit  Unit=inherit  AffineConversion=off
  mFlow_S1 : nesl_utility/PS-Simulink Converter  PhysicalDomain=network_engine_domain  SubClassName=ps_output  LeftPortType=input  RightPortType=output  PseudoPeriodic=off  Frequencies=[]  VectorFormat=inherit  Unit=inherit  AffineConversion=off
  mFraction_S1 : nesl_utility/PS-Simulink Converter  PhysicalDomain=network_engine_domain  SubClassName=ps_output  LeftPortType=input  RightPortType=output  PseudoPeriodic=off  Frequencies=[]  VectorFormat=inherit  Unit=inherit  AffineConversion=off
  relHum_S1 : nesl_utility/PS-Simulink Converter  PhysicalDomain=network_engine_domain  SubClassName=ps_output  LeftPortType=input  RightPortType=output  PseudoPeriodic=off  Frequencies=[]  VectorFormat=inherit  Unit=inherit  AffineConversion=off
  Conn1 : PMIOPort  Port=2  Side=Right
  Conn2 : PMIOPort  Side=Left
  Outport : Outport
  wires:
  aPres_S1/1 -> Bus Creator/1
  aTemp_S1/1 -> Bus Creator/2
  mFlow_S1/1 -> Bus Creator/3
  relHum_S1/1 -> Bus Creator/4
  mFraction_S1/1 -> Bus Creator/5
  MixSEnthaply_S1/1 -> Bus Creator/6
  MixDensity_S1/1 -> Bus Creator/7
  SHeat_S1/1 -> Bus Creator/8
  SEntropy_S1/1 -> Bus Creator/9
  Bus Creator/1 -> Outport/1
  connections:
  mFraction_S1/LConn1 -- Humidity & Trace Gas Sensor (MA)/RConn2
  Pressure & Temperature Sensor (MA)/RConn1 -- aPres_S1/LConn1
  mFlow_S1/LConn1 -- Flow Rate Sensor (MA)/RConn2
  Humidity & Trace Gas Sensor (MA)/LConn1 -- Pressure & Temperature Sensor (MA)/LConn1 -- Thermodynamic Properties Sensor (MA)/LConn1 -- Flow Rate Sensor (MA)/LConn1 -- Conn2/RConn1
  SEntropy_S1/LConn1 -- Thermodynamic Properties Sensor (MA)/RConn3
  aTemp_S1/LConn1 -- Pressure & Temperature Sensor (MA)/RConn2
  SHeat_S1/LConn1 -- Thermodynamic Properties Sensor (MA)/RConn4
  MixDensity_S1/LConn1 -- Thermodynamic Properties Sensor (MA)/RConn2
  MixSEnthaply_S1/LConn1 -- Thermodynamic Properties Sensor (MA)/RConn1
  relHum_S1/LConn1 -- Humidity & Trace Gas Sensor (MA)/RConn1
  Conn1/RConn1 -- Flow Rate Sensor (MA)/RConn1

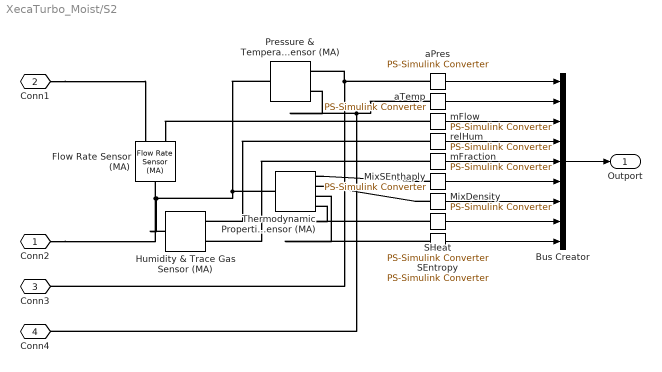
== system XecaTurbo_Moist/S2 ==
  Bus Creator : BusCreator  Inputs=9
  Flow Rate Sensor (MA) : fl_lib/Moist Air/Sensors/Flow Rate Sensor (MA)  mass_flow_measure=true  volumetric_flow_measure=false  volumetric_flow_conditions=foundation.enum.volumetric_flow_conditions.actual  p_std=0.101325 MPa  T_std=20 degC  RH_std=0.65  energy_flow_measure=false  vapor_flow_measure=false  gas_flow_measure=false
      settings: InternalSimscapePortConfiguration="{\"Bottom\":[],\"Left\":[{\"id\":\"A\",\"label\":\"A\",\"type\":\"foundation.moist_air.moist_air\"}],\"Right\":[{\"id\":\"B\",\"label\":\"B\",\"type\":\"foundation.moist_air.moist_air\"},{\"id\":\"M\",\"label\":\"M\",\"type\":\"output\"}],\"Top\":[]}"
  Humidity & Trace Gas Sensor (MA) : fl_lib/Moist Air/Sensors/Humidity & Trace Gas Sensor (MA)  moisture_on=true  moisture_spec=foundation.enum.moistureSpec.SpecificHumidity  trace_gas_on=true  trace_gas_spec=foundation.enum.trace_gas_spec.mass_fraction
      settings: InternalSimscapePortConfiguration="{\"Bottom\":[],\"Left\":[{\"id\":\"A\",\"label\":\"A\",\"type\":\"foundation.moist_air.moist_air\"}],\"Right\":[{\"id\":\"W\",\"label\":\"W\",\"type\":\"output\"},{\"id\":\"G\",\"label\":\"G\",\"type\":\"output\"}],\"Top\":[]}"
  MixDensity : nesl_utility/PS-Simulink Converter  PhysicalDomain=network_engine_domain  SubClassName=ps_output  LeftPortType=input  RightPortType=output  PseudoPeriodic=off  Frequencies=[]  VectorFormat=inherit  Unit=inherit  AffineConversion=off
  MixSEnthaply : nesl_utility/PS-Simulink Converter  PhysicalDomain=network_engine_domain  SubClassName=ps_output  LeftPortType=input  RightPortType=output  PseudoPeriodic=off  Frequencies=[]  VectorFormat=inherit  Unit=inherit  AffineConversion=off
  Pressure & Temperature Sensor (MA) : fl_lib/Moist Air/Sensors/Pressure & Temperature Sensor (MA)  reference=foundation.enum.MeasurementReference.absolute  pressure=true  pressure_spec=foundation.enum.PressureMeasementSpec.Absolute  temperature=true
      settings: InternalSimscapePortConfiguration="{\"Bottom\":[{\"id\":\"T\",\"label\":\"T\",\"type\":\"output\"}],\"Left\":[{\"id\":\"A\",\"label\":\"A\",\"type\":\"foundation.moist_air.moist_air\"}],\"Right\":[{\"id\":\"Pa\",\"label\":\"Pa\",\"type\":\"output\"}],\"Top\":[]}"
  SEntropy : nesl_utility/PS-Simulink Converter  PhysicalDomain=network_engine_domain  SubClassName=ps_output  LeftPortType=input  RightPortType=output  PseudoPeriodic=off  Frequencies=[]  VectorFormat=inherit  Unit=inherit  AffineConversion=off
  SHeat : nesl_utility/PS-Simulink Converter  PhysicalDomain=network_engine_domain  SubClassName=ps_output  LeftPortType=input  RightPortType=output  PseudoPeriodic=off  Frequencies=[]  VectorFormat=inherit  Unit=inherit  AffineConversion=off
  Thermodynamic Properties Sensor (MA) : fl_lib/Moist Air/Sensors/Thermodynamic Properties Sensor (MA)  measurement_mass_spec=foundation.enum.measurement_mass_spec.mixture  enthalpy=true  density=true  specific_heat=true  entropy=true
      settings: InternalSimscapePortConfiguration="{\"Bottom\":[{\"id\":\"CP\",\"label\":\"cp\",\"type\":\"output\"},{\"id\":\"S\",\"label\":\"s\",\"type\":\"output\"}],\"Left\":[{\"id\":\"A\",\"label\":\"A\",\"type\":\"foundation.moist_air.moist_air\"}],\"Right\":[{\"id\":\"H\",\"label\":\"h\",\"type\":\"output\"},{\"id\":\"RHO\",\"label\":\"ρ\",\"type\":\"output\"}],\"Top\":[]}"
  aPres : nesl_utility/PS-Simulink Converter  PhysicalDomain=network_engine_domain  SubClassName=ps_output  LeftPortType=input  RightPortType=output  PseudoPeriodic=off  Frequencies=[]  VectorFormat=inherit  Unit=inherit  AffineConversion=off
  aTemp : nesl_utility/PS-Simulink Converter  PhysicalDomain=network_engine_domain  SubClassName=ps_output  LeftPortType=input  RightPortType=output  PseudoPeriodic=off  Frequencies=[]  VectorFormat=inherit  Unit=inherit  AffineConversion=off
  mFlow : nesl_utility/PS-Simulink Converter  PhysicalDomain=network_engine_domain  SubClassName=ps_output  LeftPortType=input  RightPortType=output  PseudoPeriodic=off  Frequencies=[]  VectorFormat=inherit  Unit=inherit  AffineConversion=off
  mFraction : nesl_utility/PS-Simulink Converter  PhysicalDomain=network_engine_domain  SubClassName=ps_output  LeftPortType=input  RightPortType=output  PseudoPeriodic=off  Frequencies=[]  VectorFormat=inherit  Unit=inherit  AffineConversion=off
  relHum : nesl_utility/PS-Simulink Converter  PhysicalDomain=network_engine_domain  SubClassName=ps_output  LeftPortType=input  RightPortType=output  PseudoPeriodic=off  Frequencies=[]  VectorFormat=inherit  Unit=inherit  AffineConversion=off
  Conn2 : PMIOPort  Side=Left
  Conn1 : PMIOPort  Port=2  Side=Right
  Conn3 : PMIOPort  Port=3  Side=Left
  Conn4 : PMIOPort  Port=4  Side=Left
  Outport : Outport
  wires:
  aPres/1 -> Bus Creator/1
  Bus Creator/1 -> Outport/1
  relHum/1 -> Bus Creator/4
  mFraction/1 -> Bus Creator/5
  SEntropy/1 -> Bus Creator/9
  MixDensity/1 -> Bus Creator/7
  SHeat/1 -> Bus Creator/8
  mFlow/1 -> Bus Creator/3
  MixSEnthaply/1 -> Bus Creator/6
  aTemp/1 -> Bus Creator/2
  connections:
  Conn1/RConn1 -- Flow Rate Sensor (MA)/RConn1
  relHum/LConn1 -- Humidity & Trace Gas Sensor (MA)/RConn1
  MixSEnthaply/LConn1 -- Thermodynamic Properties Sensor (MA)/RConn1
  MixDensity/LConn1 -- Thermodynamic Properties Sensor (MA)/RConn2
  SHeat/LConn1 -- Thermodynamic Properties Sensor (MA)/RConn4
  aTemp/LConn1 -- Conn4/RConn1 -- Pressure & Temperature Sensor (MA)/RConn2
  SEntropy/LConn1 -- Thermodynamic Properties Sensor (MA)/RConn3
  Conn2/RConn1 -- Flow Rate Sensor (MA)/LConn1 -- Humidity & Trace Gas Sensor (MA)/LConn1 -- Thermodynamic Properties Sensor (MA)/LConn1 -- Pressure & Temperature Sensor (MA)/LConn1
  mFlow/LConn1 -- Flow Rate Sensor (MA)/RConn2
  aPres/LConn1 -- Conn3/RConn1 -- Pressure & Temperature Sensor (MA)/RConn1
  mFraction/LConn1 -- Humidity & Trace Gas Sensor (MA)/RConn2

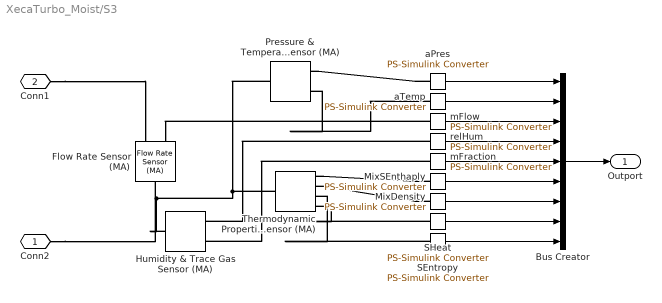
== system XecaTurbo_Moist/S3 ==
  Bus Creator : BusCreator  Inputs=9
  Flow Rate Sensor (MA) : fl_lib/Moist Air/Sensors/Flow Rate Sensor (MA)  mass_flow_measure=true  volumetric_flow_measure=false  volumetric_flow_conditions=foundation.enum.volumetric_flow_conditions.actual  p_std=0.101325 MPa  T_std=20 degC  RH_std=0.65  energy_flow_measure=false  vapor_flow_measure=false  gas_flow_measure=false
      settings: InternalSimscapePortConfiguration="{\"Bottom\":[],\"Left\":[{\"id\":\"A\",\"label\":\"A\",\"type\":\"foundation.moist_air.moist_air\"}],\"Right\":[{\"id\":\"B\",\"label\":\"B\",\"type\":\"foundation.moist_air.moist_air\"},{\"id\":\"M\",\"label\":\"M\",\"type\":\"output\"}],\"Top\":[]}"
  Humidity & Trace Gas Sensor (MA) : fl_lib/Moist Air/Sensors/Humidity & Trace Gas Sensor (MA)  moisture_on=true  moisture_spec=foundation.enum.moistureSpec.SpecificHumidity  trace_gas_on=true  trace_gas_spec=foundation.enum.trace_gas_spec.mass_fraction
      settings: InternalSimscapePortConfiguration="{\"Bottom\":[],\"Left\":[{\"id\":\"A\",\"label\":\"A\",\"type\":\"foundation.moist_air.moist_air\"}],\"Right\":[{\"id\":\"W\",\"label\":\"W\",\"type\":\"output\"},{\"id\":\"G\",\"label\":\"G\",\"type\":\"output\"}],\"Top\":[]}"
  MixDensity : nesl_utility/PS-Simulink Converter  PhysicalDomain=network_engine_domain  SubClassName=ps_output  LeftPortType=input  RightPortType=output  PseudoPeriodic=off  Frequencies=[]  VectorFormat=inherit  Unit=inherit  AffineConversion=off
  MixSEnthaply : nesl_utility/PS-Simulink Converter  PhysicalDomain=network_engine_domain  SubClassName=ps_output  LeftPortType=input  RightPortType=output  PseudoPeriodic=off  Frequencies=[]  VectorFormat=inherit  Unit=inherit  AffineConversion=off
  Pressure & Temperature Sensor (MA) : fl_lib/Moist Air/Sensors/Pressure & Temperature Sensor (MA)  reference=foundation.enum.MeasurementReference.absolute  pressure=true  pressure_spec=foundation.enum.PressureMeasementSpec.Absolute  temperature=true
      settings: InternalSimscapePortConfiguration="{\"Bottom\":[{\"id\":\"T\",\"label\":\"T\",\"type\":\"output\"}],\"Left\":[{\"id\":\"A\",\"label\":\"A\",\"type\":\"foundation.moist_air.moist_air\"}],\"Right\":[{\"id\":\"Pa\",\"label\":\"Pa\",\"type\":\"output\"}],\"Top\":[]}"
  SEntropy : nesl_utility/PS-Simulink Converter  PhysicalDomain=network_engine_domain  SubClassName=ps_output  LeftPortType=input  RightPortType=output  PseudoPeriodic=off  Frequencies=[]  VectorFormat=inherit  Unit=inherit  AffineConversion=off
  SHeat : nesl_utility/PS-Simulink Converter  PhysicalDomain=network_engine_domain  SubClassName=ps_output  LeftPortType=input  RightPortType=output  PseudoPeriodic=off  Frequencies=[]  VectorFormat=inherit  Unit=inherit  AffineConversion=off
  Thermodynamic Properties Sensor (MA) : fl_lib/Moist Air/Sensors/Thermodynamic Properties Sensor (MA)  measurement_mass_spec=foundation.enum.measurement_mass_spec.mixture  enthalpy=true  density=true  specific_heat=true  entropy=true
      settings: InternalSimscapePortConfiguration="{\"Bottom\":[{\"id\":\"CP\",\"label\":\"cp\",\"type\":\"output\"},{\"id\":\"S\",\"label\":\"s\",\"type\":\"output\"}],\"Left\":[{\"id\":\"A\",\"label\":\"A\",\"type\":\"foundation.moist_air.moist_air\"}],\"Right\":[{\"id\":\"H\",\"label\":\"h\",\"type\":\"output\"},{\"id\":\"RHO\",\"label\":\"ρ\",\"type\":\"output\"}],\"Top\":[]}"
  aPres : nesl_utility/PS-Simulink Converter  PhysicalDomain=network_engine_domain  SubClassName=ps_output  LeftPortType=input  RightPortType=output  PseudoPeriodic=off  Frequencies=[]  VectorFormat=inherit  Unit=inherit  AffineConversion=off
  aTemp : nesl_utility/PS-Simulink Converter  PhysicalDomain=network_engine_domain  SubClassName=ps_output  LeftPortType=input  RightPortType=output  PseudoPeriodic=off  Frequencies=[]  VectorFormat=inherit  Unit=inherit  AffineConversion=off
  mFlow : nesl_utility/PS-Simulink Converter  PhysicalDomain=network_engine_domain  SubClassName=ps_output  LeftPortType=input  RightPortType=output  PseudoPeriodic=off  Frequencies=[]  VectorFormat=inherit  Unit=inherit  AffineConversion=off
  mFraction : nesl_utility/PS-Simulink Converter  PhysicalDomain=network_engine_domain  SubClassName=ps_output  LeftPortType=input  RightPortType=output  PseudoPeriodic=off  Frequencies=[]  VectorFormat=inherit  Unit=inherit  AffineConversion=off
  relHum : nesl_utility/PS-Simulink Converter  PhysicalDomain=network_engine_domain  SubClassName=ps_output  LeftPortType=input  RightPortType=output  PseudoPeriodic=off  Frequencies=[]  VectorFormat=inherit  Unit=inherit  AffineConversion=off
  Conn2 : PMIOPort  Side=Left
  Conn1 : PMIOPort  Port=2  Side=Right
  Outport : Outport
  wires:
  aTemp/1 -> Bus Creator/2
  aPres/1 -> Bus Creator/1
  SEntropy/1 -> Bus Creator/9
  MixSEnthaply/1 -> Bus Creator/6
  MixDensity/1 -> Bus Creator/7
  mFraction/1 -> Bus Creator/5
  mFlow/1 -> Bus Creator/3
  relHum/1 -> Bus Creator/4
  Bus Creator/1 -> Outport/1
  SHeat/1 -> Bus Creator/8
  connections:
  mFraction/LConn1 -- Humidity & Trace Gas Sensor (MA)/RConn2
  aPres/LConn1 -- Pressure & Temperature Sensor (MA)/RConn1
  mFlow/LConn1 -- Flow Rate Sensor (MA)/RConn2
  Pressure & Temperature Sensor (MA)/LConn1 -- Thermodynamic Properties Sensor (MA)/LConn1 -- Humidity & Trace Gas Sensor (MA)/LConn1 -- Flow Rate Sensor (MA)/LConn1 -- Conn2/RConn1
  SEntropy/LConn1 -- Thermodynamic Properties Sensor (MA)/RConn3
  aTemp/LConn1 -- Pressure & Temperature Sensor (MA)/RConn2
  SHeat/LConn1 -- Thermodynamic Properties Sensor (MA)/RConn4
  MixDensity/LConn1 -- Thermodynamic Properties Sensor (MA)/RConn2
  MixSEnthaply/LConn1 -- Thermodynamic Properties Sensor (MA)/RConn1
  relHum/LConn1 -- Humidity & Trace Gas Sensor (MA)/RConn1
  Conn1/RConn1 -- Flow Rate Sensor (MA)/RConn1
